simulink model "control_structure_dA"  (R2015a)
settings: Solver=ode45  StartTime=0.0  StopTime=10.0  RelTol=1e-3
values from neighbouring files (symbols this model uses):
  A_r = 0.1    [example_transient_response.m]    (also in lag_network_example_1.m = 0; lag_network_example_2.m = 1; lag_network_example_3.m = 0; lead_network_example_2.m = 0)
libraries: cstblocks x1
settings Model: Creator=Riccardo  LastModifiedBy=Riccardo

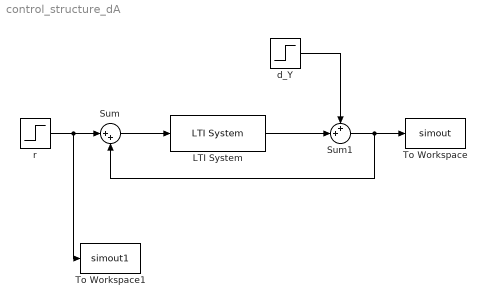
== system control_structure_dA ==
  LTI System : cstblocks/LTI System  sys=L3  IC=[]
  Sum : Sum  Inputs=|++
  Sum1 : Sum  Inputs=++|
  To Workspace : ToWorkspace  VariableName=simout  SaveFormat=Timeseries  SampleTime=-1
  To Workspace1 : ToWorkspace  VariableName=simout1  SaveFormat=Timeseries  SampleTime=-1
  "d_Y " : Step  SampleTime=0
  "r " : Step  Time=0  After=A_r  SampleTime=0
  wires:
  "r "/1 -> To Workspace1/1, Sum/1
  Sum/1 -> LTI System/1
  Sum1/1 -> Sum/2, To Workspace/1
  LTI System/1 -> Sum1/2
  "d_Y "/1 -> Sum1/1
